simulink model "mpc_controller"  (R2024b)
settings: Solver=VariableStepAuto  StartTime=0.0  StopTime=20  RelTol=1e-3
values from neighbouring files (symbols this model uses):
  Iz = 1960    [mpc3.m]    (also in prueba_mpc.m; prueba_mpc2.m)
  lf = 1.177    [mpc3.m]    (also in prueba_mpc.m; prueba_mpc2.m)
  lr = 1.358    [mpc3.m]    (also in prueba_mpc.m; prueba_mpc2.m)
  m = 1400    [mpc3.m]    (also in prueba_mpc.m; prueba_mpc2.m)
  vx = 10    [mpc3.m]    (also in prueba_mpc.m; prueba_mpc2.m)
undefined symbols (not defined in the file or in its folder): miu, steering_angle
libraries: mpclib x1
settings Model: Creator=inaki  LastModifiedBy=inaki

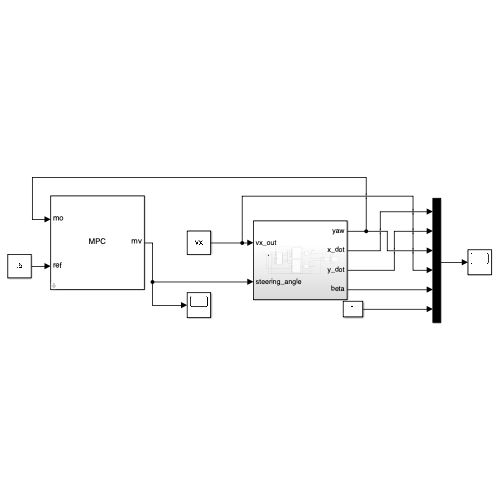
[thumbnail: Simulink's stored preview of the top-level diagram]
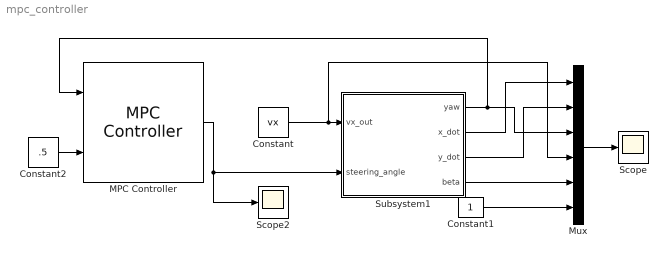
== system mpc_controller ==
  Constant : Constant  Value=vx
  Constant1 : Constant
  Constant2 : Constant  Value=.5
  MPC Controller : mpclib/MPC Controller  SCDEnableBlockLinearizationSpecification=on  mpcobj=mpc1  is_multiple=0  enable_value=0  return_u0=off  updateMPCinCallerWorkspace=on  md_inport=off  mv_inport=off  uref_inport=off  return_cost=off  return_mvseq=off  return_qpstatus=off  return_xseq=off  return_state=off  return_ovseq=off  state_inport=off  umin_inport=off  umax_inport=off  ymin_inport=off  ymax_inport=off  cc_inport=off  ywt_inport=off  uwt_inport=off  duwt_inport=off  rhoeps_inport=off  pm_inport=off  MaximumP=10  HorizonChoice=FixedHorizon  n_ts=0.1  n_p=10  n_mv=1  n_md=0  n_ud=0  n_mo=1  n_uo=0  BlockDataType=double  SampleTimeInherited=off  switch_inport=off
  Mux : Mux  Inputs=6
  Scope : Scope
  Scope2 : Scope
  Subsystem1 : Subsystem
  wires:
  Constant/1 -> Mux/4, Subsystem1/1(vx_out)
  MPC Controller/1 -> Scope2/1, Subsystem1/2(steering_angle)
  Subsystem1/1(yaw) -> MPC Controller/1, Mux/3
  Subsystem1/2(x_dot) -> Mux/1
  Subsystem1/3(y_dot) -> Mux/2
  Subsystem1/4(beta) -> Mux/5
  Constant1/1 -> Mux/6
  Constant2/1 -> MPC Controller/2
  Mux/1 -> Scope/1

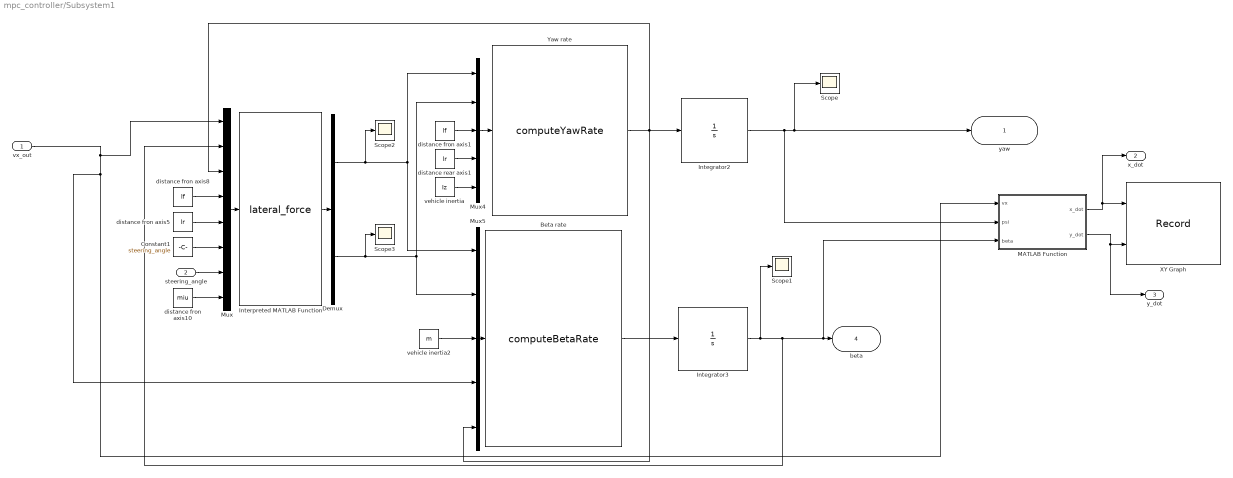
== system mpc_controller/Subsystem1 ==
  vx_out : Inport
  steering_angle : Inport  Port=2
  Beta rate : MATLABFcn  MATLABFcn=computeBetaRate
  Constant1 : Constant  Value=steering_angle
  Demux : Demux  Outputs=2
  Integrator2 : Integrator
  Integrator3 : Integrator
  Interpreted MATLAB Function : MATLABFcn  MATLABFcn=lateral_force  OutputDimensions=2
  MATLAB Function : MATLAB Function  TreatAsAtomicUnit=on
  Mux : Mux  Inputs=8
  Mux4 : Mux  Inputs=5
  Mux5 : Mux  Inputs=5
  Scope{,1..3} (4 alike) : Scope
  XY Graph : Record  FileSettingsInternal="{\"entries\":[{\"content\":{\"excelSettings\":{\"content\":{},\"type\":\"Streamout.ExcelSettings\"}},\"type\":\"Streamout.FileSettingStorage\",\"uuid\":\"\"}],\"packageUris\":[\"http:\\/\\/schema.mathworks.com\\/mf0\\/streamout_blocks\\/R2020a\"],\"version\":\"1.0\"}"  Layout=[1 1]  SignalsInternal="{\"entries\":[{\"content\":{\"signals\":[{\"content\":{\"blockPath\":[],\"dimensions\":[1],\"domain\":\"\",\"lineColor\":\"#a2142f\",\"plots\":[ 1 ],\"port\":1,\"signalID\":1,\"signalName\":\"MATLAB Function:1\"},\"type\":\"RecordBlkView.Signal\",\"uuid\":\"\"},{\"content\":{\"blockPath\":[],\"dimensions\":[1],\"domain\":\"\",\"lineColor\":\"#139fff\",\"plots\":[ 1 ],\"port\":2,\"signalID\":2,\"signalName\":\"MATLAB Function:2\"},\"type\":\"RecordBlkView.Signal\",\"uuid\":\"\"}]},\"type\":\"RecordBlkView.InputSignals\",\"uuid\":\"\"}],\"packageUris\":[\"http:\\/\\/schema.mathworks.com\\/mf0\\/streamout_blocks\\/R2020a\"],\"version\":\"1.0\"}"  VisualizationBindings="{\"xyplotplugin\":{\"info\":[{\"series\":[{\"bindingParametersList\":[{\"parameter\":\"X-Axis\",\"signalID\":1,\"signalName\":\"MATLAB Function:1\"},{\"parameter\":\"Y-Axis\",\"signalID\":2,\"signalName\":\"MATLAB Function:2\"}],\"seriesID\":0}],\"subplotID\":1}]}}"  CompatibilityTag=XY
  Yaw rate : MATLABFcn  MATLABFcn=computeYawRate
  distance fron axis1 : Constant  Value=lf
  distance fron axis10 : Constant  Value=miu
  distance fron axis5 : Constant  Value=lr
  distance fron axis8 : Constant  Value=lf
  distance rear axis1 : Constant  Value=lr
  vehicle inertia : Constant  Value=Iz
  vehicle inertia2 : Constant  Value=m
  yaw : Outport
  x_dot : Outport  Port=2
  y_dot : Outport  Port=3
  beta : Outport  Port=4
  wires:
  distance fron axis10/1 -> Mux/8
  distance fron axis8/1 -> Mux/4
  distance fron axis5/1 -> Mux/5
  Constant1/1 -> Mux/6
  steering_angle/1 -> Mux/7
  Demux/1 -> Scope2/1, Mux5/1, Mux4/1
  Demux/2 -> Scope3/1, Mux5/2, Mux4/2
  vehicle inertia2/1 -> Mux5/3
  Integrator2/1 -> MATLAB Function/2(psi), Scope/1, yaw/1
  Mux4/1 -> Yaw rate/1
  distance rear axis1/1 -> Mux4/4
  distance fron axis1/1 -> Mux4/3
  vehicle inertia/1 -> Mux4/5
  Interpreted MATLAB Function/1 -> Demux/1
  Mux/1 -> Interpreted MATLAB Function/1
  Mux5/1 -> Beta rate/1
  Beta rate/1 -> Integrator3/1
  Yaw rate/1 -> Mux/3, Mux5/5, Integrator2/1
  Integrator3/1 -> MATLAB Function/3(beta), beta/1, Mux/2, Scope1/1
  vx_out/1 -> Mux5/4, MATLAB Function/1(vx), Mux/1
  MATLAB Function/1(x_dot) -> x_dot/1, XY Graph/1
  MATLAB Function/2(y_dot) -> y_dot/1, XY Graph/2

== matlab function mpc_controller/Subsystem1/MATLAB Function ==
  data: vx input; psi input; x_dot output; beta input; y_dot output
function [x_dot,y_dot] = computeVehiclePosition(vx,psi,beta) 
    vy = vx * tan(beta);
    x_dot = vx * cos(psi) - vy * sin(psi); 
    y_dot = vx * sin(psi) + vy * cos(psi); 

   
end
